simulink model "Model1111"  (R2014a)
settings: Solver=ode45  StartTime=0.0  StopTime=10.0  RelTol=1e-3
values from neighbouring files (symbols this model uses):
  Bs = 1    [Parameters.m]    (also in matlab_Kad.mat)
  l = 0.201061929829747    (= 0.20106192983)    [Parameters.m]
  omega = 2*pi*50    (= 314.159265359)    [Parameters.m]    (also in matlab_Kad.mat)
  r = 5000    [Parameters.m]    (also in matlab_Kad.mat)
  R0 = 0.225000000000000    (= 0.225)    [Parameters.m]    (also in matlab_Kad.mat)
  S = h*(d1-d2)/2    (= 0.0001875)    [Calc_hysteresis.m]    (also in Parameters.m = 0.000425; matlab_Kad.mat = 0.000425)
  w1 = 1    [Calc_hysteresis.m]    (also in Parameters.m; matlab_Kad.mat)
  w2 = 10    [Calc_hysteresis.m]    (also in Parameters.m = 120; matlab_Kad.mat = 120)
libraries: simulink x1
settings Model: Creator=Андрей  LastModifiedBy=Андрей

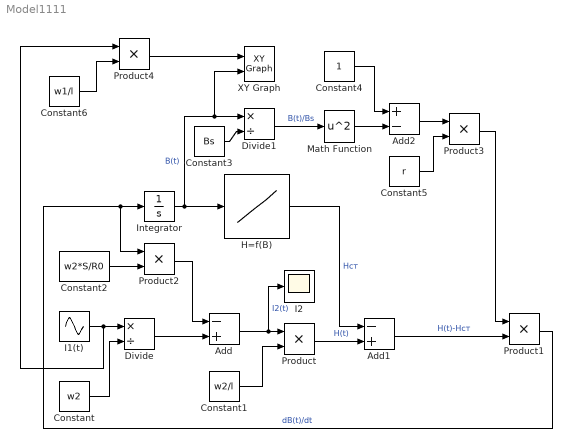
== system Model1111 ==
  Add : Sum  Inputs=-+
  Add1 : Sum  Inputs=-+
  Add2 : Sum  Inputs=+-
  Constant : Constant  Value=w2
  Constant1 : Constant  Value=w2/l
  Constant2 : Constant  Value=w2*S/R0
  Constant3 : Constant  Value=Bs
  Constant4 : Constant
  Constant5 : Constant  Value=r
  Constant6 : Constant  Value=w1/l
  Divide : Product  Inputs=*/
  Divide1 : Product  Inputs=*/
  H=f(B) : Lookup_n-D  NumberOfTableDimensions=1  BreakpointsForDimension1=[-5:5]  Table=tanh([-5:5])  InternalRulePriority=Speed  RndMeth=Simplest  InputSameDT=on
  I1(t) : Sin  Frequency=omega  SampleTime=0
  I2 : Scope
  Integrator : Integrator
  Math Function : Math  Operator=square  SaturateOnIntegerOverflow=on
  Product{,1..4} (5 alike) : Product
  XY Graph : simulink/Sinks/XY Graph  xmin=-1  xmax=1  ymin=-1  ymax=1  st=-1
  wires:
  I1(t)/1 -> Product4/1, Divide/1
  Constant/1 -> Divide/2
  Divide/1 -> Add/2
  Add/1 -> Product/1, I2/1  "I2(t)"
  Constant1/1 -> Product/2
  Product/1 -> Add1/2  "H(t)"
  Add1/1 -> Product1/2  "H(t)-Hст"
  Product1/1 -> Product2/1, Integrator/1  "dB(t)/dt"
  Constant2/1 -> Product2/2
  Product2/1 -> Add/1
  Integrator/1 -> XY Graph/2, Divide1/1, H=f(B)/1  "B(t)"
  H=f(B)/1 -> Add1/1  "Hст"
  Constant3/1 -> Divide1/2
  Divide1/1 -> Math Function/1  "B(t)/Bs"
  Add2/1 -> Product3/1
  Constant5/1 -> Product3/2
  Product3/1 -> Product1/1
  Math Function/1 -> Add2/2
  Constant4/1 -> Add2/1
  Product4/1 -> XY Graph/1
  Constant6/1 -> Product4/2
